simulink model "error1234"  (R2013a)
settings: Solver=ode45  StartTime=0.0  StopTime=T  RelTol=1e-3
undefined symbols (not defined in the file or in its folder): K, Set_point1, Set_point2
libraries: simulink x1
settings Model: Creator=srinivasan  LastModifiedBy=srinivasan

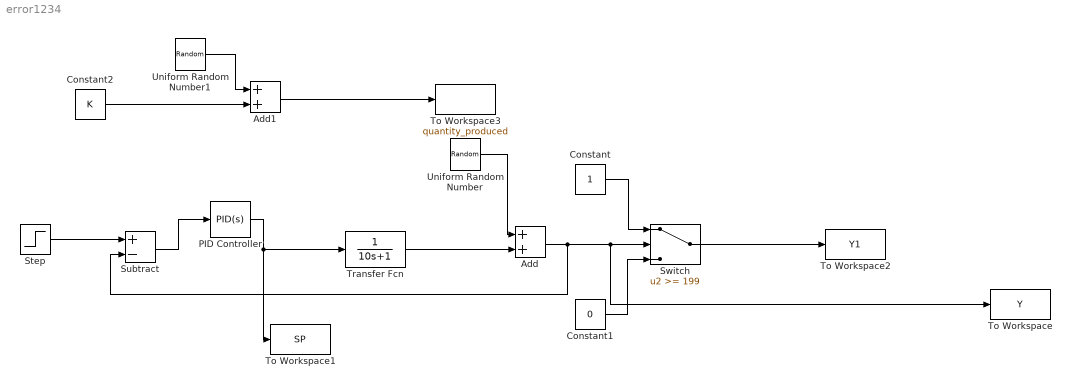
== system error1234 ==
  Add : Sum
  Add1 : Sum
  Constant : Constant
  Constant1 : Constant  Value=0
  Constant2 : Constant  Value=K
  PID Controller : simulink/Continuous/PID Controller  Controller=PID  TimeDomain=Continuous-time  SampleTime=1  IntegratorMethod=Forward Euler  FilterMethod=Forward Euler  Form=Ideal  P=1  I=1  D=0  N=0  InitialConditionSource=internal  InitialConditionForIntegrator=0  InitialConditionForFilter=0  ExternalReset=none  LimitOutput=off  UpperSaturationLimit=inf  LowerSaturationLimit=-inf  LinearizeAsGain=on  AntiWindupMode=none  Kb=1  TrackingMode=off  Kt=1  PParamMin=[]  PParamMax=[]  IParamMin=[]  IParamMax=[]  DParamMin=[]  DParamMax=[]  NParamMin=[]  NParamMax=[]  KbParamMin=[]  KbParamMax=[]  KtParamMin=[]  KtParamMax=[]  POutMin=[]  POutMax=[]  IOutMin=[]  IOutMax=[]  IOutDataTypeStr=double  DOutMin=[]  DOutMax=[]  DOutDataTypeStr=double  NOutMin=[]  NOutMax=[]  KbOutMin=[]  KbOutMax=[]  KtOutMin=[]  KtOutMax=[]  IntegratorOutMin=[]  IntegratorOutMax=[]  FilterOutMin=[]  FilterOutMax=[]  SumOutMin=[]  SumOutMax=[]  SumI1OutMin=[]  SumI1OutMax=[]  SumI2OutMin=[]  SumI2OutMax=[]  SumI3OutMin=[]  SumI3OutMax=[]  SumDOutMin=[]  SumDOutMax=[]  SaturationOutMin=[]  SaturationOutMax=[]  IntegratorContinuousStateAttributes=''  IntegratorStateMustResolveToSignalObject=off  IntegratorRTWStateStorageClass=Auto  FilterContinuousStateAttributes=''  FilterStateMustResolveToSignalObject=off  FilterRTWStateStorageClass=Auto
  Step : Step  Time=100  Before=Set_point1  After=Set_point2  SampleTime=0
  Subtract : Sum  Inputs=+-
  Switch : Switch  Threshold=199
  To Workspace : ToWorkspace  VariableName=Y  SampleTime=1  SaveFormat=Timeseries
  To Workspace1 : ToWorkspace  VariableName=SP  SampleTime=-1  SaveFormat=Timeseries
  To Workspace2 : ToWorkspace  VariableName=Y1  SampleTime=1  SaveFormat=Timeseries
  To Workspace3 : ToWorkspace  VariableName=quantity_produced  SampleTime=1  SaveFormat=Timeseries
  Transfer Fcn : TransferFcn  Denominator=[10 1]
  Uniform Random Number : UniformRandomNumber  SampleTime=0.1
  Uniform Random Number1 : UniformRandomNumber  SampleTime=0.1
  wires:
  Step/1 -> Subtract/1
  Transfer Fcn/1 -> Add/2
  Uniform Random Number/1 -> Add/1
  Add/1 -> Subtract/2, To Workspace/1, Switch/2
  Constant/1 -> Switch/1
  Constant1/1 -> Switch/3
  Subtract/1 -> PID Controller/1
  PID Controller/1 -> Transfer Fcn/1, To Workspace1/1
  Switch/1 -> To Workspace2/1
  Constant2/1 -> Add1/2
  Uniform Random Number1/1 -> Add1/1
  Add1/1 -> To Workspace3/1
